simulink model "fec_prototype_03"  (R2013a)
settings: Solver=FixedStepDiscrete  SolverMode=SingleTasking  StartTime=0.0  StopTime=inf  RelTol=1e-3
PreLoadFcn:
  | maxNumErrs = 100;
  | maxNumBits = 1e6;
  | EbNo = 4;
InitFcn:
  | ;
StartFcn:
  | ;
StopFcn:
  | ;
undefined symbols (not defined in the file or in its folder): commblksprivate, Info
libraries: commdigbbndpm3 x2, commcnvcod2 x2, dspquant2 x1, commchan3 x1, commrandsrc2 x1, commsink2 x1
PreSaveFcn:
  | ;
CloseFcn:
  | ;
settings Model: MinMaxOverflowLogging=MinMaxAndOverflow  Creator=The MathWorks Inc.  LastModifiedBy=lifesatrip
settings DataIOCC: SignalLoggingSaveFormat=ModelDataLogs  SignalLogging=off  SaveTime=off
settings OptimizationCC: InlineParams=on  ExpressionDepthLimit=2147483647  LocalBlockOutputs=off  InitFltsAndDblsToZero=on  OptimizeModelRefInitCode=on  LifeSpan=1
settings DebuggingCC: SaveWithParameterizedLinksMsg=none  SignalResolutionControl=TryResolveAllWithWarning  MultiTaskDSMMsg=warning  MultiTaskCondExecSysMsg=none  FcnCallInpInsideContextMsg=UseLocalSettings  StrictBusMsg=Warning
settings HardwareCC: ProdBitPerInt=16  ProdIntDivRoundTo=Floor  ProdEndianess=LittleEndian  ProdWordSize=16  ProdHWDeviceType=16-bit Generic  TargetEndianess=LittleEndian  TargetHWDeviceType=MATLAB Host  ProdEqTarget=off
settings RTWCC: SystemTargetFile=ert.tlc  TemplateMakefile=ert_default_tmf  Description=Real-Time Workshop Embedded Coder (no auto configuration)  GenerateReport=on  RetainRTWFile=on  ProcessScript=ert_make_rtw_hook  IncludeHyperlinkInReport=on  LaunchReport=on  IncludeERTFirstTime=on
settings CodeAppCC: CustomSymbolStrType=$N$R$M  InternalIdentifier=Classic
settings ERTTargetCC: TargetFcnLib=ansi_tfl_tmw.mat  SupportAbsoluteTime=off  MatFileLogging=on  ERTCustomFileTemplate=example_file_process.tlc

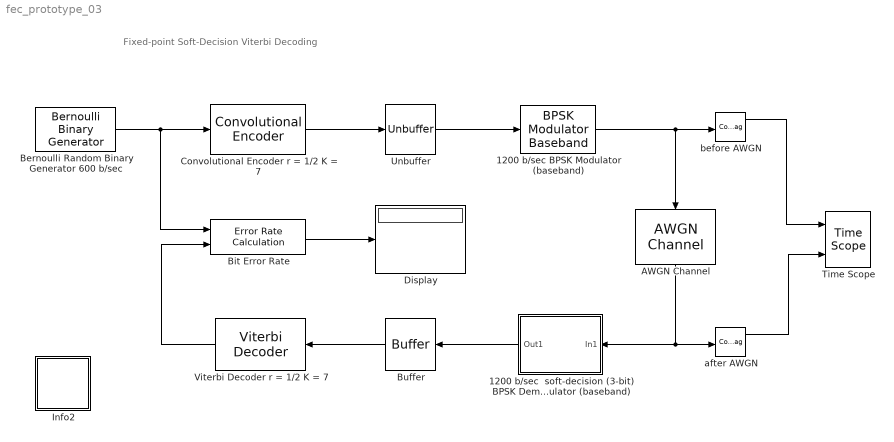
== system fec_prototype_03 ==
  note: Fixed-point Soft-Decision Viterbi Decoding
  1200 b/sec  soft-decision (3-bit) BPSK Demodulator (baseband) : Subsystem
  1200 b/sec BPSK Modulator (baseband) : commdigbbndpm3/BPSK Modulator Baseband  Ph=0  outDtype=double  outWordLen=16  outUDDataType=sfix(16)  outFracLenMode=Best precision  outFracLen=15
  AWGN Channel : commchan3/AWGN Channel  InputProcessing=Columns as channels (frame based)  seed=113  noiseMode="Signal to noise ratio  (Eb/No)"  EbNodB=EbNo - 10*log10(2)  EsNodB=1  SNRdB=10  bitsPerSym=1  Ps=1  Tsym=1/1200  variance=(1*0.005)/((1/200)*10^(EbNo/10))
  Bernoulli Random Binary Generator 600 b/sec : commrandsrc2/Bernoulli Binary Generator  P=0.5  seed=911  Ts=1/600  frameBased=on  sampPerFrame=1  orient=off  outDataType=boolean
  Bit Error Rate : commsink2/Error Rate Calculation  N=49  st_delay=0  cp_mode=Entire frame  subframe=[]  PMode=Port  WsName=ErrorVec  RsMode2=off  stop=off  numErr=maxNumErrs  maxBits=maxNumBits
  Buffer : Buffer  N=2  TreatMby1Signals=One channel
  Convolutional Encoder r = 1/2 K = 7 : commcnvcod2/Convolutional Encoder  trellis=poly2trellis(7, [171 133])  opMode=Continuous  DelayedResetAction=off  hasIniStPort=off  hasFinStPort=off  usePuncVector=off  punctureVector=[1; 1; 0; 1; 0; 1]  reset=Unused parameter value
  Display : Display
  Info2 : Subsystem  AncestorBlock=commblksprivate/Info  mask(Info){}
      settings: OpenFcn=helpview([docroot '/toolbox/comm/comm.map'], 'doc_fixpt_vitsoftdec')
      mask Display: disp('Info')
  Time Scope : TimeScope  NumInputPorts=2  DefaultConfigurationName=spbscopes.TimeScopeBlockCfg
      settings: CopyFcn=scopeextensions.ScopeBlock.callback(gcbh, 'onBlockCopy', gcbh);  DeleteFcn=scopeextensions.ScopeBlock.callback(gcbh, 'onBlockDelete');  PreSaveFcn=scopeextensions.ScopeBlock.callback(gcbh, 'onModelSave');  NameChangeFcn=scopeextensions.ScopeBlock.callback(gcbh, 'onBlockRename');  CloseFcn=scopeextensions.ScopeBlock.callback(gcbh, 'onBlockClose');  PreDeleteFcn=scopeextensions.ScopeBlock.callback(gcbh, 'onBlockPreDelete');
  Unbuffer : Unbuffer  SampleBasedProcessing=Same as frame based
  Viterbi Decoder r = 1/2 K = 7 : commcnvcod2/Viterbi Decoder  trellis=poly2trellis(7, [171 133])  isPunctured=off  punctureVector=[1; 1; 0; 1; 0; 1]  erasures=off  dectype=Soft decision  runSigValErrCheck=off  nsdecb=3  smWordLength=16  tbdepth=48  opmode=Continuous  reset=off  outDataType=boolean  delayedResetAction=off
  after AWGN : ComplexToRealImag
  before AWGN : ComplexToRealImag
  wires:
  Bernoulli Random Binary Generator 600 b/sec/1 -> Convolutional Encoder r = 1/2 K = 7/1, Bit Error Rate/1
  Bit Error Rate/1 -> Display/1
  Viterbi Decoder r = 1/2 K = 7/1 -> Bit Error Rate/2
  Convolutional Encoder r = 1/2 K = 7/1 -> Unbuffer/1
  Unbuffer/1 -> 1200 b/sec BPSK Modulator (baseband)/1
  Buffer/1 -> Viterbi Decoder r = 1/2 K = 7/1
  1200 b/sec  soft-decision (3-bit) BPSK Demodulator (baseband)/1(Out1) -> Buffer/1
  1200 b/sec BPSK Modulator (baseband)/1 -> AWGN Channel/1, before AWGN/1
  AWGN Channel/1 -> 1200 b/sec  soft-decision (3-bit) BPSK Demodulator (baseband)/1(In1), after AWGN/1
  after AWGN/1 -> Time Scope/2
  before AWGN/1 -> Time Scope/1

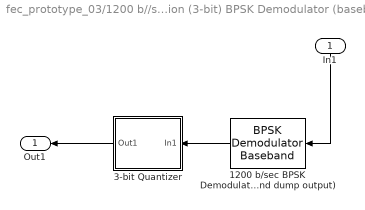
== system fec_prototype_03/1200 b//sec  soft-decision (3-bit) BPSK Demodulator (baseband) ==
  In1 : Inport
  " 3-bit Quantizer" : Subsystem
  1200 b/sec BPSK Demodulatonr (integrate and dump output) : commdigbbndpm3/BPSK Demodulator Baseband  Ph=0  DecType=Log-likelihood ratio  VarSource=Dialog  Variance=1/(10^((EbNo-10*log10(2))/10))  outDtype=double  derotateFactorWordLen=16
  Out1 : Outport
  wires:
  " 3-bit Quantizer"/1(Out1) -> Out1/1
  In1/1 -> 1200 b/sec BPSK Demodulatonr (integrate and dump output)/1
  1200 b/sec BPSK Demodulatonr (integrate and dump output)/1 -> " 3-bit Quantizer"/1(In1)

== system fec_prototype_03/Info2 ==

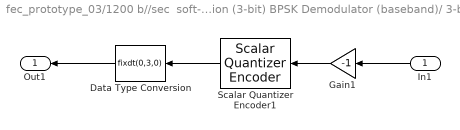
== system fec_prototype_03/1200 b//sec  soft-decision (3-bit) BPSK Demodulator (baseband)/ 3-bit Quantizer ==
  In1 : Inport
  Data Type Conversion : DataTypeConversion  OutDataTypeStr=fixdt(0,3,0)
  Gain1 : Gain  Gain=-1
  Scalar Quantizer Encoder1 : dspquant2/Scalar Quantizer Encoder  paramSrc=Specify via dialog  partType=Unbounded  BBoundary=[-6:2:6]/4  UBoundary=[-3:3]  SearchMethod=Linear  tieBreakRule=Choose the higher index  outQU=off  outQError=off  codebook=[1.5:9.5]  outStatus=off  invalidin=Clip  idtype=uint8  roundingMode=Floor  overflowMode=off
  Out1 : Outport
  wires:
  In1/1 -> Gain1/1
  Data Type Conversion/1 -> Out1/1
  Scalar Quantizer Encoder1/1 -> Data Type Conversion/1
  Gain1/1 -> Scalar Quantizer Encoder1/1
